simulink model "discreto"  (R2013a)
settings: Solver=ode45  StartTime=0.0  StopTime=10.0  RelTol=1e-3
values from neighbouring files (symbols this model uses):
  hdis = hdis'    [Ejercicio1.m]    (also in ejercicioDiscreto.m)
  kidis = ktdis(1,3)    [Ejercicio1.m]    (also in ejercicioDiscreto.m)
  kpdis = ktdis(1,1:2)    [Ejercicio1.m]    (also in ejercicioDiscreto.m)
undefined symbols (not defined in the file or in its folder): adis, bdis, cdis
settings Model: Creator=tp.aulas4  LastModifiedBy=tp.aulas4

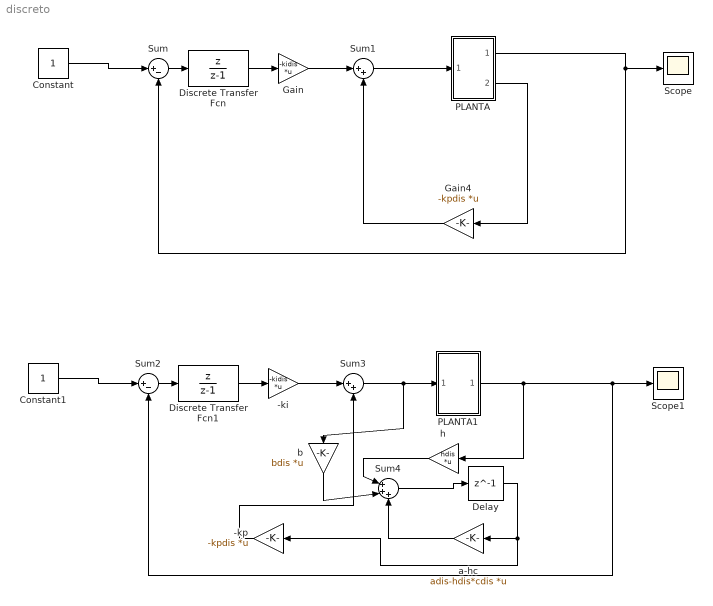
== system discreto ==
  "-ki " : Gain  Gain=-kidis  Multiplication=Matrix(K*u) (u vector)  SampleTime=0.1
  -kp : Gain  Gain=-kpdis  Multiplication=Matrix(K*u) (u vector)  SampleTime=0.1
  Constant : Constant  SampleTime=0.1
  Constant1 : Constant  SampleTime=0.1
  Delay : Delay  DelayLength=1  SampleTime=0.1
  Discrete Transfer Fcn : DiscreteTransferFcn  Numerator=[1 0]  Denominator=[1 -1]  SampleTime=0.1
  Discrete Transfer Fcn1 : DiscreteTransferFcn  Numerator=[1 0]  Denominator=[1 -1]  SampleTime=0.1
  Gain : Gain  Gain=-kidis  Multiplication=Matrix(K*u) (u vector)  SampleTime=0.1
  Gain4 : Gain  Gain=-kpdis  Multiplication=Matrix(K*u) (u vector)  SampleTime=0.1
  PLANTA : Subsystem
  PLANTA1 : Subsystem
  Scope : Scope
  Scope1 : Scope
  Sum : Sum  Inputs=|+-  SampleTime=0.1
  Sum1 : Sum  Inputs=|++  SampleTime=0.1
  Sum2 : Sum  Inputs=|+-  SampleTime=0.1
  Sum3 : Sum  Inputs=|++  SampleTime=0.1
  Sum4 : Sum  Inputs=|+++  SampleTime=0.1
  a-hc : Gain  Gain=adis-hdis*cdis  Multiplication=Matrix(K*u) (u vector)  SampleTime=0.1
  b : Gain  Gain=bdis  Multiplication=Matrix(K*u) (u vector)  SampleTime=0.1
  h : Gain  Gain=hdis  Multiplication=Matrix(K*u) (u vector)  SampleTime=0.1
  wires:
  Gain/1 -> Sum1/1
  Gain4/1 -> Sum1/2
  Constant/1 -> Sum/1
  PLANTA/1(Out1) -> Sum/2, Scope/1
  Sum1/1 -> PLANTA/1(In1)
  PLANTA/2(Out2) -> Gain4/1
  "-ki "/1 -> Sum3/1
  Constant1/1 -> Sum2/1
  Sum3/1 -> PLANTA1/1(In1), b/1
  h/1 -> Sum4/1
  b/1 -> Sum4/2
  a-hc/1 -> Sum4/3
  -kp/1 -> Sum3/2
  Sum/1 -> Discrete Transfer Fcn/1
  Discrete Transfer Fcn/1 -> Gain/1
  PLANTA1/1(Out1) -> h/1, Sum2/2, Scope1/1
  Sum2/1 -> Discrete Transfer Fcn1/1
  Discrete Transfer Fcn1/1 -> "-ki "/1
  Sum4/1 -> Delay/1
  Delay/1 -> -kp/1, a-hc/1

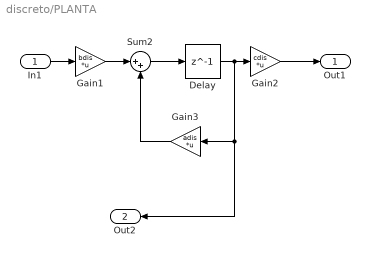
== system discreto/PLANTA ==
  In1 : Inport
  Delay : Delay  DelayLength=1
  Gain1 : Gain  Gain=bdis  Multiplication=Matrix(K*u) (u vector)  SampleTime=0.1
  Gain2 : Gain  Gain=cdis  Multiplication=Matrix(K*u) (u vector)  SampleTime=0.1
  Gain3 : Gain  Gain=adis  Multiplication=Matrix(K*u) (u vector)  SampleTime=0.1
  Sum2 : Sum  Inputs=|++  SampleTime=0.1
  Out1 : Outport
  Out2 : Outport  Port=2
  wires:
  Delay/1 -> Out2/1, Gain3/1, Gain2/1
  In1/1 -> Gain1/1
  Gain1/1 -> Sum2/1
  Gain3/1 -> Sum2/2
  Gain2/1 -> Out1/1
  Sum2/1 -> Delay/1

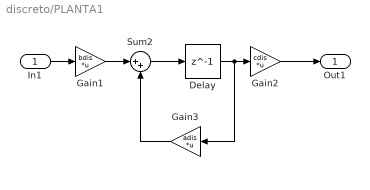
== system discreto/PLANTA1 ==
  In1 : Inport
  Delay : Delay  DelayLength=1
  Gain1 : Gain  Gain=bdis  Multiplication=Matrix(K*u) (u vector)  SampleTime=0.1
  Gain2 : Gain  Gain=cdis  Multiplication=Matrix(K*u) (u vector)  SampleTime=0.1
  Gain3 : Gain  Gain=adis  Multiplication=Matrix(K*u) (u vector)  SampleTime=0.1
  Sum2 : Sum  Inputs=|++  SampleTime=0.1
  Out1 : Outport
  wires:
  Delay/1 -> Gain3/1, Gain2/1
  In1/1 -> Gain1/1
  Gain1/1 -> Sum2/1
  Gain3/1 -> Sum2/2
  Gain2/1 -> Out1/1
  Sum2/1 -> Delay/1
